simulink model "projekat1_PID_init"  (R2018a)
settings: Solver=ode4  StartTime=0.0  StopTime=100000.0  FixedStep=0.1  RelTol=1e-3
values from neighbouring files (symbols this model uses):
  Ca = 10^-6    (= 1e-06)    [projekat1.m]
  Cb = 10^-6    (= 1e-06)    [projekat1.m]
  Fa = 0.016667    [projekat1.m]
  kw = 10^-14    (= 1e-14)    [projekat1.m]
  uep = eval (ue)    [projekat1.m]
  V = 30    [projekat1.m]
settings Model: Creator=svorc  LastModifiedBy=svorc
settings DataIOCC: ReturnWorkspaceOutputs=on
settings DebuggingCC: SFMachineParentedDataDiag=error
settings SFSimCC: SimUseLocalCustomCode=on
settings RTWCC: RTWUseLocalCustomCode=on

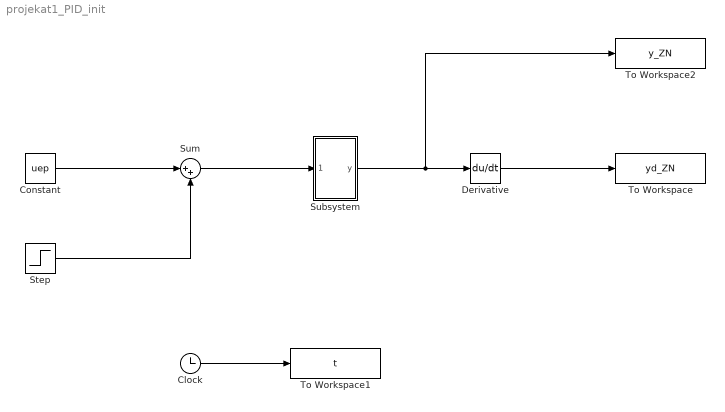
== system projekat1_PID_init ==
  Clock : Clock
  Constant : Constant  Value=uep
  Derivative : Derivative
  Step : Step  Time=10000  After=0.1*uep  SampleTime=0
  Subsystem : Subsystem
  Sum : Sum  Inputs=|++
  To Workspace : ToWorkspace  VariableName=yd_ZN  SampleTime=-1
  To Workspace1 : ToWorkspace  VariableName=t  SampleTime=-1
  To Workspace2 : ToWorkspace  VariableName=y_ZN  SampleTime=-1
  wires:
  Sum/1 -> Subsystem/1(Input)
  Constant/1 -> Sum/1
  Step/1 -> Sum/2
  Subsystem/1(y) -> To Workspace2/1, Derivative/1
  Derivative/1 -> To Workspace/1
  Clock/1 -> To Workspace1/1

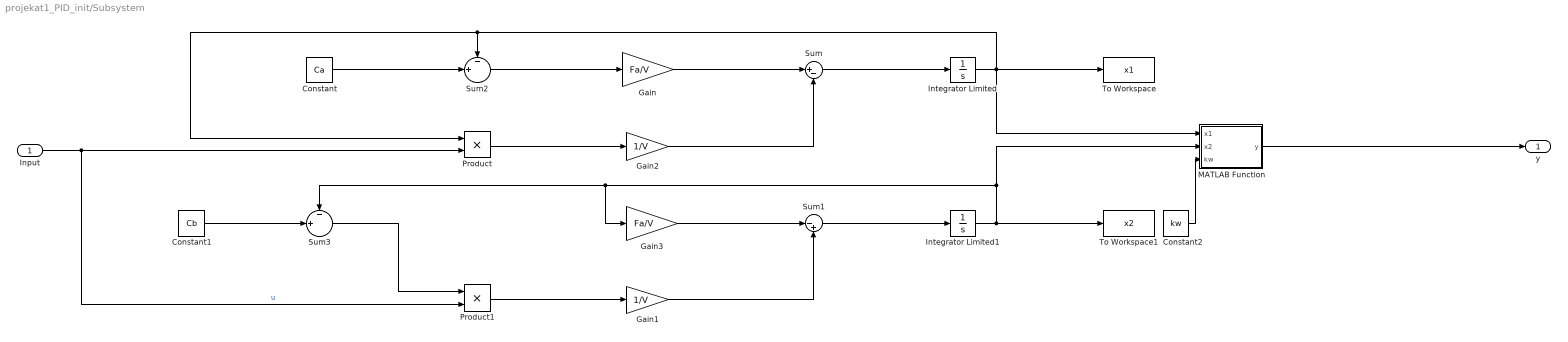
== system projekat1_PID_init/Subsystem ==
  Input : Inport
  Constant : Constant  Value=Ca
  Constant1 : Constant  Value=Cb
  Constant2 : Constant  Value=kw
  Gain : Gain  Gain=Fa/V
  Gain1 : Gain  Gain=1/V
  Gain2 : Gain  Gain=1/V
  Gain3 : Gain  Gain=Fa/V
  Integrator Limited : Integrator  InitialCondition=Ca  LimitOutput=on  UpperSaturationLimit=Ca  LowerSaturationLimit=0
  Integrator Limited1 : Integrator  LimitOutput=on  UpperSaturationLimit=Cb  LowerSaturationLimit=0
  MATLAB Function : MATLAB Function  TreatAsAtomicUnit=on
  Product : Product
  Product1 : Product
  Sum : Sum  Inputs=|+-
  Sum1 : Sum  Inputs=|-+
  Sum2 : Sum  Inputs=-|+||
  Sum3 : Sum  Inputs=-|+||
  To Workspace : ToWorkspace  VariableName=x1  SampleTime=-1
  To Workspace1 : ToWorkspace  VariableName=x2  SampleTime=-1
  y : Outport
  wires:
  Sum3/1 -> Product1/1
  Sum/1 -> Integrator Limited/1
  Gain/1 -> Sum/1
  Input/1 -> Product/2, Product1/2  "u"
  Gain3/1 -> Sum1/1
  Integrator Limited1/1 -> MATLAB Function/2(x2), Gain3/1, Sum3/1, To Workspace1/1
  Integrator Limited/1 -> To Workspace/1, MATLAB Function/1(x1), Sum2/1, Product/1
  Constant1/1 -> Sum3/2
  Sum1/1 -> Integrator Limited1/1
  Product1/1 -> Gain1/1
  Constant/1 -> Sum2/2
  Gain2/1 -> Sum/2
  MATLAB Function/1(y) -> y/1
  Gain1/1 -> Sum1/2
  Product/1 -> Gain2/1
  Sum2/1 -> Gain/1
  Constant2/1 -> MATLAB Function/3(kw)

== matlab function projekat1_PID_init/Subsystem/MATLAB Function ==
  data: x1 input; y output; x2 input; kw input
function y = fcn(x1, x2, kw)

y = -log10(sqrt((x2-x1)^2 / 4 + kw) - (x2 - x1) / 2);
